simulink model "PNEUMA"  (R2023b)
settings: Solver=ode23tb  StartTime=0  StopTime=3600  FixedStep=0.001  MaxStep=time_step_new  RelTol=0.01  EnableMultiTasking=on
values from neighbouring files (symbols this model uses):
  A = 20.9    [Gas_Exchange_IC.m]    (also in getPneumonia.m = (LF1-LF2)/(1-exp(Rresolve*(t2(end)-t2(1)))))
  a1 = 0.3836    [Dissociation_Spencer_IC.m]    (also in Gas_Exchange_IC.m; Respiratory_IC.m)
  a2 = 1.819    [Dissociation_Spencer_IC.m]    (also in Gas_Exchange_IC.m; Respiratory_IC.m)
  alpha1 = 0.02598    [Dissociation_Spencer_IC.m]    (also in Gas_Exchange_IC.m; Respiratory_IC.m)
  alpha2 = 0.05591    [Dissociation_Spencer_IC.m]    (also in Gas_Exchange_IC.m; Respiratory_IC.m)
  B = 92.8    [Gas_Exchange_IC.m]    (also in getPneumonia.m = LungFunction(end)-A)
  beta1 = 0.012275    [Dissociation_Spencer_IC.m]    (also in Gas_Exchange_IC.m; Respiratory_IC.m)
  beta2 = 0.03255    [Dissociation_Spencer_IC.m]    (also in Gas_Exchange_IC.m; Respiratory_IC.m)
  C = 10570    [Gas_Exchange_IC.m]
  C1 = 9    [Dissociation_Spencer_IC.m]    (also in Gas_Exchange_IC.m; Respiratory_IC.m)
  C2 = 87.00    (= 87)    [Dissociation_Spencer_IC.m]    (also in Gas_Exchange_IC.m; Respiratory_IC.m)
  Circadian_Period = 24    [Respiratory_IC.m]    (also in State_UA_Khoo_IC.m)
  CvCO2IC = 0.5116    [Body_Khoo_IC.m]    (also in Gas_Exchange_IC.m; Respiratory_IC.m = 0.5247)
  CvO2IC = 0.1672    [Body_Khoo_IC.m]    (also in Gas_Exchange_IC.m; Respiratory_IC.m = 0.1639)
  D = -5.251    [Gas_Exchange_IC.m]
  Dead1CO2IC = 0.1020    (= 0.102)    [Dead_Space_Khoo_IC.m]    (also in Gas_Exchange_IC.m; Respiratory_IC.m = 39.5616)
  Dead1O2IC = 149.8824    [Dead_Space_Khoo_IC.m]    (also in Gas_Exchange_IC.m; Respiratory_IC.m = 104.3637)
  Dead2CO2IC = 0.5274    [Dead_Space_Khoo_IC.m]    (also in Gas_Exchange_IC.m; Respiratory_IC.m = 39.6736)
  Dead2O2IC = 149.3923    [Dead_Space_Khoo_IC.m]    (also in Gas_Exchange_IC.m; Respiratory_IC.m = 104.2258)
  Dead3CO2IC = 2.2996    [Dead_Space_Khoo_IC.m]    (also in Gas_Exchange_IC.m; Respiratory_IC.m = 39.8127)
  Dead3O2IC = 147.3503    [Dead_Space_Khoo_IC.m]    (also in Gas_Exchange_IC.m; Respiratory_IC.m = 104.0505)
  Dead4CO2IC = 8.2293    [Dead_Space_Khoo_IC.m]    (also in Gas_Exchange_IC.m; Respiratory_IC.m = 40.0061)
  Dead4O2IC = 140.5179    [Dead_Space_Khoo_IC.m]    (also in Gas_Exchange_IC.m; Respiratory_IC.m = 103.8005)
  Dead5CO2IC = 22.0757    [Dead_Space_Khoo_IC.m]    (also in Gas_Exchange_IC.m; Respiratory_IC.m = 40.3359)
  Dead5O2IC = 124.5641    [Dead_Space_Khoo_IC.m]    (also in Gas_Exchange_IC.m; Respiratory_IC.m = 103.3579)
  DtotalIC = 0.3    [NeuroMuscular_IC.m]    (also in Respiratory_IC.m = 0.32)
  E_CW = 5    [Pleural_Schuessler_IC.m]    (also in Pmus_Flow_Younes_IC.m; Resp_Mech_IC.m; Respiratory_IC.m)
  E_L = 5    [Pleural_Schuessler_IC.m]    (also in Pmus_Flow_Younes_IC.m; Resp_Mech_IC.m; Respiratory_IC.m)
  fc = 0.4/60    (= 0.00666666666667)    [Respiratory_IC.m]    (also in State_UA_Khoo_IC.m)
  fcs_max = 47.78    [Cardiovascular_IC.m]    (also in Reflex_Ursino_IC.m)
  fcs_min = 2.52    [Cardiovascular_IC.m]    (also in Reflex_Ursino_IC.m)
  fcs_zero = 25    [Respiratory_IC.m]
  FlowIC = 0    [Pmus_Flow_Younes_IC.m]    (also in Resp_Mech_IC.m; Respiratory_IC.m)
  fp_inf = 6.3    [Respiratory_IC.m]
  fp_zero = 3.2    [Respiratory_IC.m]
  fs_inf = 2.10    (= 2.1)    [Respiratory_IC.m]
  fs_zero = 16.11    [Respiratory_IC.m]
  ftbs_min = 0.1    [Cardiovascular_IC.m]    (also in SA_Node_Ursino_IC.m)
  gc = 0.008/60    (= 0.000133333333333)    [Respiratory_IC.m]    (also in State_UA_Khoo_IC.m)
  h = 0.0183    [Brain_Khoo_IC.m]    (also in Gas_Exchange_IC.m; Respiratory_IC.m)
  HP_basal = 0.58    [Cardiovascular_IC.m]    (also in SA_Node_Ursino_IC.m)
  Ic = 45    [Gas_Exchange_IC.m]    (also in Respiratory_IC.m; Vent_Drive_Khoo_IC.m)
  IpCO2 = 38    [Gas_Exchange_IC.m]    (also in Respiratory_IC.m; Vent_Drive_Khoo_IC.m)
  IpO2 = 102.4    [Gas_Exchange_IC.m]    (also in Respiratory_IC.m; Vent_Drive_Khoo_IC.m)
  K1 = 13    [Dissociation_Spencer_IC.m]    (also in Gas_Exchange_IC.m; Respiratory_IC.m)
  K2 = 194.4    [Dissociation_Spencer_IC.m]    (also in Gas_Exchange_IC.m; Respiratory_IC.m)
  k_cs = 11.758    [Cardiovascular_IC.m]    (also in Reflex_Ursino_IC.m)
  k_p = 7.06    [Respiratory_IC.m]
  k_s = 0.07    [Respiratory_IC.m]
  lambda = 863    [Gas_Exchange_IC.m]    (also in Lungs_Khoo_IC.m; Respiratory_IC.m)
  Mech_Vent_pressure = 17    [Mech_vent_test.m]
  MRbCO2 = 0.0517    [Brain_Khoo_IC.m]    (also in Gas_Exchange_IC.m; Respiratory_IC.m)
  MRCO2 = 0.0033    [Body_Khoo_IC.m]    (also in Gas_Exchange_IC.m; Respiratory_IC.m)
  MRO2 = 0.0038    [Body_Khoo_IC.m]    (also in Gas_Exchange_IC.m; Respiratory_IC.m)
  NM_block_gain = 1    [Mech_vent_test.m]
  PACO2_delayIC = 39.6041    [Cardio_Mix_Lange_IC.m]    (also in Gas_Exchange_IC.m; Respiratory_IC.m = 40.4448)
  PaCO2firstIC = 0.2150    (= 0.215)    [Cardio_Mix_Lange_IC.m]    (also in Gas_Exchange_IC.m; Respiratory_IC.m = -0.2465)
  PACO2IC = 37.1484    [Gas_Exchange_IC.m]    (also in Lungs_Khoo_IC.m; Respiratory_IC.m = 40.9432)
  PaCO2secondIC = 38.4577    [Cardio_Mix_Lange_IC.m]    (also in Gas_Exchange_IC.m; Respiratory_IC.m = 40.3928)
  PAO2_delayIC = 103.8436    [Cardio_Mix_Lange_IC.m]    (also in Gas_Exchange_IC.m; Respiratory_IC.m = 103.1223)
  PaO2firstIC = -0.2838    [Cardio_Mix_Lange_IC.m]    (also in Gas_Exchange_IC.m; Respiratory_IC.m = 0.3557)
  PAO2IC = 107.1983    [Gas_Exchange_IC.m]    (also in Lungs_Khoo_IC.m; Respiratory_IC.m = 102.5153)
  PaO2secondIC = 105.4828    [Cardio_Mix_Lange_IC.m]    (also in Gas_Exchange_IC.m; Respiratory_IC.m = 103.1435)
  PbCO2IC = 48.2858    [Brain_Khoo_IC.m]    (also in Gas_Exchange_IC.m; Respiratory_IC.m = 48.5383)
  PICO2 = 0    [Dead_Space_Khoo_IC.m]    (also in Gas_Exchange_IC.m; Respiratory_IC.m)
  PIO2 = 150    [Dead_Space_Khoo_IC.m]    (also in Gas_Exchange_IC.m; Respiratory_IC.m)
  PIO2_change = -90    [Mech_vent_test.m]    (also in Respiratory_IC.m = 0)
  Pn = 90    [Cardiovascular_IC.m]    (also in Reflex_Ursino_IC.m)
  Pt_frcIC1 = 0    [Pmus_Flow_Younes_IC.m]    (also in Resp_Mech_IC.m; Respiratory_IC.m)
  Pt_frcIC2 = 0    [Pmus_Flow_Younes_IC.m]    (also in Resp_Mech_IC.m; Respiratory_IC.m)
  QdBo = 0.8333    [Brain_Khoo_IC.m]    (also in Gas_Exchange_IC.m; Respiratory_IC.m)
  R_AW = 1.27    [Pleural_Schuessler_IC.m]    (also in Pmus_Flow_Younes_IC.m; Resp_Mech_IC.m; Respiratory_IC.m)
  R_CW = 1.03    [Pleural_Schuessler_IC.m]    (also in Pmus_Flow_Younes_IC.m; Resp_Mech_IC.m; Respiratory_IC.m)
  R_L = 1.69    [Pleural_Schuessler_IC.m]    (also in Pmus_Flow_Younes_IC.m; Resp_Mech_IC.m; Respiratory_IC.m)
  RC = 0.06    [Pleural_Schuessler_IC.m]    (also in Pmus_Flow_Younes_IC.m; Resp_Mech_IC.m; Respiratory_IC.m)
  rc = 0.2/60    (= 0.00333333333333)    [Respiratory_IC.m]    (also in State_UA_Khoo_IC.m)
  SbCO2 = 0.3600    (= 0.36)    [Brain_Khoo_IC.m]    (also in Gas_Exchange_IC.m; Respiratory_IC.m)
  SCO2 = 0.0043    [Brain_Khoo_IC.m]    (also in Gas_Exchange_IC.m; Respiratory_IC.m)
  SWAo = 0.007    [Respiratory_IC.m]    (also in State_UA_Khoo_IC.m)
  T1 = 1    [Cardio_Mix_Lange_IC.m]    (also in Gas_Exchange_IC.m; Respiratory_IC.m)
  T2 = 2    [Cardio_Mix_Lange_IC.m]    (also in Gas_Exchange_IC.m; Respiratory_IC.m)
  t_end_new = 4*24*60*60    (= 345600)    [Mech_vent_test.m]
  t_end_UA = 0    [Respiratory_IC.m]    (also in State_UA_Khoo_IC.m)
  t_Mech_Vent_duration = 0    [Mech_vent_test.m]
  t_Mech_Vent_start = 0    [Mech_vent_test.m]
  t_Mueller_duration = 0    [NeuroMuscular_IC.m]
  t_Mueller_insp = 0    [NeuroMuscular_IC.m]
  t_Mueller_start = 0    [NeuroMuscular_IC.m]
  t_NM_block_duration = 0    [Mech_vent_test.m]
  t_NM_block_start = 0    [Mech_vent_test.m]
  t_O2_duration = 0    [Mech_vent_test.m]    (also in Respiratory_IC.m)
  t_O2_start = 0    [Mech_vent_test.m]    (also in Respiratory_IC.m)
  t_start_new = 0    [Mech_vent_test.m]
  t_start_UA = 0    [Respiratory_IC.m]    (also in State_UA_Khoo_IC.m)
  t_valsalva_duration = 0    [NeuroMuscular_IC.m]
  t_valsalva_insp = 0    [NeuroMuscular_IC.m]
  t_valsalva_start = 0    [NeuroMuscular_IC.m]
  time_step = time_step    [acquire_data.m]    (also in acquire_data_save.m)
  VC = 5    [Pmus_Flow_Younes_IC.m]    (also in Resp_Mech_IC.m; Respiratory_IC.m)
  Vdead1 = 0.03    [Dead_Space_Khoo_IC.m]    (also in Gas_Exchange_IC.m; Respiratory_IC.m)
  Vdead2 = 0.03    [Dead_Space_Khoo_IC.m]    (also in Gas_Exchange_IC.m; Respiratory_IC.m)
  Vdead3 = 0.03    [Dead_Space_Khoo_IC.m]    (also in Gas_Exchange_IC.m; Respiratory_IC.m)
  Vdead4 = 0.03    [Dead_Space_Khoo_IC.m]    (also in Gas_Exchange_IC.m; Respiratory_IC.m)
  Vdead5 = 0.03    [Dead_Space_Khoo_IC.m]    (also in Gas_Exchange_IC.m; Respiratory_IC.m)
  Ventilator_rate = 12    [Mech_vent_test.m]
  VTCO2 = 15    [Body_Khoo_IC.m]    (also in Gas_Exchange_IC.m; Respiratory_IC.m)
  VtIC = 0    [Pmus_Flow_Younes_IC.m]    (also in Resp_Mech_IC.m; Respiratory_IC.m)
  VTO2 = 6    [Body_Khoo_IC.m]    (also in Gas_Exchange_IC.m; Respiratory_IC.m)
  Z = 0.0227    [Dissociation_Spencer_IC.m]    (also in Gas_Exchange_IC.m; Respiratory_IC.m)
undefined symbols (not defined in the file or in its folder): A_0_ua, alpha_E_FFA_Heart, alpha_E_FFA_muscle, alpha_E_GLC_Heart, alpha_E_GLC_muscle, alpha_E_GLY_muscle, alpha_E_PYR_muscle, alpha_E_TGL_adipose, alpha_E_TGL_GI, alpha_E_TGL_Heart, alpha_E_TGL_muscle, Arousal_UAIC, C_ua_awake, Cbp, Cbv, Ce_0, Cep, Cev, Chp, Chv, Cla, Clamp_class, Cmp, Cmv, Cpa, CPAP_pressure, Cpp, Cpv, Cra, Csa, Csp, Csv, CvbO2_n, CvhO2_n, CvmO2_n, DAY, delay, DietBlock, Dx, Fb, fchemo_max, fchemo_min, fchemoIC, flsIC, Ftas_I0, ftas_min, ftas_r0, FVC_activation, gain_E, Gamma, Gas_sleep, Gas_sleepM, Gb, Gblock, GbO2, Gbs_sleep, gcc_sa, gcc_sb, gcc_sp, Gclamp ... (+144)
libraries: simulink x4, dspstat3 x4, simulink_extras x2
(part 2 of 8)

== system PNEUMA/Cardiovascular System/Right Heart ==
  note: Right Heart
  note: Vura (Right Atrium Unstressed Volume)
      | Vurv (Right Ventricle Unstressed Volume)
      | Vrv (Right Ventricle Volume)
      | Vra (Right Atrium Volume)
      | Pra (Right Atrium Pressure)
      | Prv (Right Ventricle Pressure)
      | Qra (Flow into Right Atrium)
      | Qir (Flow into Right Ventricle)
      | Qor (Flow out of Right Ventricle)
      | LHeart (Left Ventricle Function)
  In1 : Inport
  CHF Gain : Gain
  CHF Gain1 : Gain
  Constant2 : Constant  Value=Vura
  Constant3 : Constant  Value=Vurv
  Gain : Gain  Gain=1/Cra  SaturateOnIntegerOverflow=on  OutDataTypeStr=Inherit: Same as input  ParamDataTypeStr=Inherit: Same as input
  Gain2 : Gain  Gain=1/Rra  SaturateOnIntegerOverflow=on  OutDataTypeStr=Inherit: Same as input  ParamDataTypeStr=Inherit: Same as input
  Integrator : Integrator
  Integrator1 : Integrator
  Pmaxrv--Ppa ---------------------- Rrv : Subsystem
  Product : Product  RndMeth=Zero
  SubSystem : Subsystem
  SubSystem1 : Subsystem
  Sum : Sum  Inputs=|+-  InputSameDT=on  SaturateOnIntegerOverflow=on  OutDataTypeStr=Inherit: Same as first input
  Sum1 : Sum  Inputs=|+-  InputSameDT=on  SaturateOnIntegerOverflow=on  OutDataTypeStr=Inherit: Same as first input
  Sum2 : Sum  Inputs=|++
  Sum3 : Sum  Inputs=+-  InputSameDT=on  SaturateOnIntegerOverflow=on  OutDataTypeStr=Inherit: Same as first input
  Sum4 : Sum  Inputs=+-  InputSameDT=on  SaturateOnIntegerOverflow=on  OutDataTypeStr=Inherit: Same as first input
  Sum6 : Sum  Inputs=|++
  Switch2 : Switch
  pulmonary valve : Saturate  UpperLimit=inf  LowerLimit=0
  tricuspid valve : Saturate  UpperLimit=inf  LowerLimit=0
  Out1 : Outport
  tag scope: Pra=scoped, Vra=scoped, Vrv=scoped, Wrv=scoped
  wires:
  In1/1 -> Sum/1  "Qra"
  Sum/1 -> Integrator/1
  [Ppa] -> Sum1/2
  Gain2/1 -> Sum/2, Sum4/1  "Qir"
  Integrator/1 -> SubSystem/2(+)
  Constant2/1 -> SubSystem/1(_)
  SubSystem1/1(Out) -> [Vrv]
  SubSystem/1(Out) -> Gain/1, [Vra]
  Constant3/1 -> SubSystem1/1(_)
  Integrator1/1 -> SubSystem1/2(+)
  Sum1/1 -> pulmonary valve/1, Switch2/2
  [Ppa] -> Switch2/1
  tricuspid valve/1 -> CHF Gain1/1
  pulmonary valve/1 -> Pmaxrv--Ppa ---------------------- Rrv/2(P)  "Qor"
  Pmaxrv--Ppa ---------------------- Rrv/1(Flow) -> CHF Gain/1  "Qor"
  [RHeart] -> Switch2/3, Pmaxrv--Ppa ---------------------- Rrv/1(Pmax), Sum1/1  "Pmaxrv"
  Sum4/1 -> Integrator1/1, Product/2
  Sum3/1 -> tricuspid valve/1
  Gain/1 -> Sum6/1  "Pra"
  Sum6/1 -> [Pra], Sum3/1
  Switch2/1 -> Sum2/2, Product/1  "Prv"
  Sum2/1 -> Sum3/2
  [gPpl] -> Sum2/1, Sum6/2
  Product/1 -> [Wrv]
  CHF Gain/1 -> Out1/1, Sum4/2
  CHF Gain1/1 -> Gain2/1

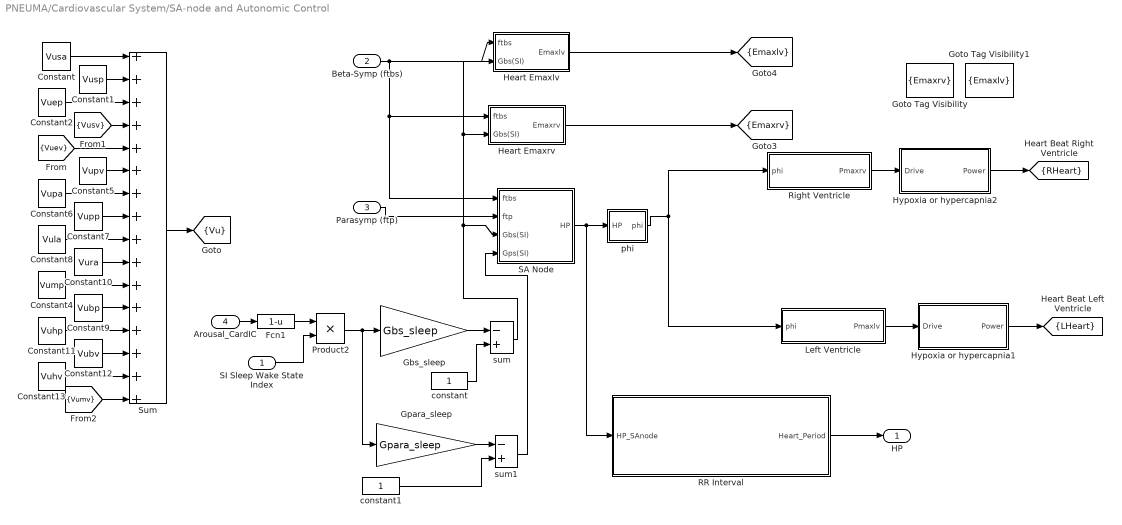
== system PNEUMA/Cardiovascular System/SA-node and Autonomic Control ==
  SI Sleep Wake State Index : Inport
  Beta-Symp (ftbs) : Inport  Port=2
  Parasymp (ftp) : Inport  Port=3
  Arousal_CardIC : Inport  Port=4
  Constant : Constant  Value=Vusa
  Constant1 : Constant  Value=Vusp
  Constant10 : Constant  Value=Vura
  Constant11 : Constant  Value=Vuhp
  Constant12 : Constant  Value=Vubv
  Constant13 : Constant  Value=Vuhv
  Constant2 : Constant  Value=Vuep
  Constant4 : Constant  Value=Vump
  Constant5 : Constant  Value=Vupv
  Constant6 : Constant  Value=Vupa
  Constant7 : Constant  Value=Vupp
  Constant8 : Constant  Value=Vula
  Constant9 : Constant  Value=Vubp
  Fcn1 : Fcn  Expr=1-u
  Gbs_sleep : Gain  Gain=Gbs_sleep  SaturateOnIntegerOverflow=on  OutDataTypeStr=Inherit: Same as input  ParamDataTypeStr=Inherit: Same as input
  Goto Tag Visibility : GotoTagVisibility  GotoTag=Emaxrv
  Goto Tag Visibility1 : GotoTagVisibility  GotoTag=Emaxlv
  Gpara_sleep : Gain  Gain=Gpara_sleep  SaturateOnIntegerOverflow=on  OutDataTypeStr=Inherit: Same as input  ParamDataTypeStr=Inherit: Same as input
  Heart Emaxlv : Subsystem
  Heart Emaxrv : Subsystem
  Hypoxia or hypercapnia1 : Subsystem
  Hypoxia or hypercapnia2 : Subsystem
  Left Ventricle : Subsystem
  Product2 : Product  InputSameDT=on  SaturateOnIntegerOverflow=on  OutDataTypeStr=Inherit: Same as first input
  RR Interval : Subsystem
  Right Ventricle : Subsystem
  SA Node : Subsystem
  Sum : Sum  Inputs=++++++++++++++++  InputSameDT=on  SaturateOnIntegerOverflow=on  OutDataTypeStr=Inherit: Same as first input
  constant : Constant
  constant1 : Constant
  phi : Subsystem
  sum : Sum  Inputs=-+  InputSameDT=on  SaturateOnIntegerOverflow=on  OutDataTypeStr=Inherit: Same as first input
  sum1 : Sum  Inputs=-+  InputSameDT=on  SaturateOnIntegerOverflow=on  OutDataTypeStr=Inherit: Same as first input
  HP : Outport
  tag scope: Emaxlv=scoped, Emaxrv=scoped, LHeart=scoped, RHeart=scoped, Vu=scoped
  wires:
  Arousal_CardIC/1 -> Fcn1/1
  SI Sleep Wake State Index/1 -> Product2/2
  sum/1 -> Heart Emaxrv/2(Gbs(SI)), Heart Emaxlv/2(Gbs(SI)), SA Node/3(Gbs(SI))
  sum1/1 -> SA Node/4(Gps(SI))
  Fcn1/1 -> Product2/1
  Product2/1 -> Gbs_sleep/1, Gpara_sleep/1
  Gbs_sleep/1 -> sum/1
  constant/1 -> sum/2
  Gpara_sleep/1 -> sum1/1
  constant1/1 -> sum1/2
  Sum/1 -> [Vu]
  Constant/1 -> Sum/1
  Constant2/1 -> Sum/3
  Constant1/1 -> Sum/2
  [Vusv] -> Sum/4
  [Vuev] -> Sum/5
  Constant5/1 -> Sum/6
  Constant6/1 -> Sum/7
  Constant7/1 -> Sum/8
  Constant8/1 -> Sum/9
  Constant10/1 -> Sum/10
  Constant4/1 -> Sum/11
  Constant9/1 -> Sum/12
  Constant11/1 -> Sum/13
  Constant12/1 -> Sum/14
  Constant13/1 -> Sum/15
  [Vumv] -> Sum/16
  phi/1(phi) -> Right Ventricle/1(phi), Left Ventricle/1(phi)
  SA Node/1(HP) -> phi/1(HP), RR Interval/1(HP_SAnode)
  Beta-Symp (ftbs)/1 -> Heart Emaxrv/1(ftbs), SA Node/1(ftbs), Heart Emaxlv/1(ftbs)
  Parasymp (ftp)/1 -> SA Node/2(ftp)
  RR Interval/1(Heart_Period) -> HP/1
  Heart Emaxlv/1(Emaxlv) -> [Emaxlv]
  Heart Emaxrv/1(Emaxrv) -> [Emaxrv]
  Left Ventricle/1(Pmaxlv) -> Hypoxia or hypercapnia1/1(Drive)
  Hypoxia or hypercapnia1/1(Power) -> [LHeart]
  Right Ventricle/1(Pmaxrv) -> Hypoxia or hypercapnia2/1(Drive)
  Hypoxia or hypercapnia2/1(Power) -> [RHeart]

== system PNEUMA/Cardiovascular System/Systemic ==
  note: Psa (Systemic Arteries Pressure)
      | Psp (Splanchnic Peripheral Pressure)
      | Pep (Extrasplanchnic Peripheral Pressure)
      | Psv (Splanchnic Venous Pressure)
      | Pvc (Vena Cava Pressure)
      | Pra (Right Atrium Pressure)
      | For (Flow from Left Heart)
      | Fsa (Flow to Systemic Aorta)
      | Fil (Flow to Left Atrium)
      | Fvc (Flow to Vena Cava)
      | Fra (Flow to Right Atrium)
      | Vusa (Systemic Arteries Unstressed Volume)
      | Vusp (Extrasplanchnic Venous Unstressed Volume)
      | Vuep (Splanchnic Venous Unstressed Volume)
      | Vuev (Extrasplanchnic Venous Unstressed Volume)
      | Vusv (Splanchnic Venous Unstressed Volume)
  note: Systemic Circulation
  Qlv : Inport
  Goto Tag Visibility7 : GotoTagVisibility  GotoTag=Vvc
  Systemic Arteries : Subsystem
  Systemic Peripheral & Venous Circulation : Subsystem
  Vena Cava : Subsystem
  Qra : Outport
  Qmp : Outport  Port=2
  Qbp : Outport  Port=3
  Qhp : Outport  Port=4
  wires:
  Qlv/1 -> Systemic Arteries/1(Qlv)  "Fol"
  Systemic Arteries/1(Qsa) -> Systemic Peripheral & Venous Circulation/1(Qsa)
  Vena Cava/1(Qra) -> Qra/1
  Systemic Peripheral & Venous Circulation/1(Qvc) -> Vena Cava/1(Qvc)
  Systemic Peripheral & Venous Circulation/2(Qmp) -> Qmp/1
  Systemic Peripheral & Venous Circulation/3(Qbp) -> Qbp/1
  Systemic Peripheral & Venous Circulation/4(Qhp) -> Qhp/1

== system PNEUMA/Cardiovascular System/TPR Change ==
  Alpha Symp (ftas) : Inport
  Alpha Symp (ftas_vein) : Inport  Port=2
  AI (arousal  Index) : Inport  Port=3
  "SI (Sleep Index) " : Inport  Port=4
  Fcn1 : Fcn  Expr=1-u
  Gas_sleep : Gain  Gain=Gas_sleep  SaturateOnIntegerOverflow=on  OutDataTypeStr=Inherit: Same as input  ParamDataTypeStr=Inherit: Same as input
  Math Function{,1..4} (5 alike) : Math  Operator=reciprocal  SignedPower=on
  Mux : Mux  Inputs=10
  Peri Circ Rep : Subsystem
  Peri Circ Rmp : Subsystem
  Peri Circ Rsp : Subsystem
  Product2 : Product  InputSameDT=on  SaturateOnIntegerOverflow=on  OutDataTypeStr=Inherit: Same as first input
  Saving TPR : Subsystem
  Sum1 : Sum  Inputs=+++++  InputSameDT=on  SaturateOnIntegerOverflow=on  OutDataTypeStr=Inherit: Same as first input
  Sum3 : Sum  Inputs=-+  InputSameDT=on  SaturateOnIntegerOverflow=on  OutDataTypeStr=Inherit: Same as first input
  Venous Circ Vuev : Subsystem
  Venous Circ Vumv : Subsystem
  Venous Circ Vusv : Subsystem
  constant : Constant
  tag scope: Rep=scoped, Rmpn=scoped, Rsp=scoped, TPR_change=global, Vuev=scoped, Vumv=scoped, Vusv=scoped
  wires:
  AI (arousal  Index)/1 -> Fcn1/1
  "SI (Sleep Index) "/1 -> Product2/2
  Fcn1/1 -> Product2/1
  Product2/1 -> Gas_sleep/1
  constant/1 -> Sum3/2
  Gas_sleep/1 -> Sum3/1
  Peri Circ Rep/1(Rep) -> [Rep], Math Function1/1, Mux/2  "Rep"
  Venous Circ Vusv/1(Vusv) -> [Vusv], Mux/7  "Vusv"
  Venous Circ Vuev/1(Vuev) -> [Vuev], Mux/8  "Vuev"
  Peri Circ Rsp/1(Rsp) -> [Rsp], Math Function/1, Mux/1  "Rsp"
  Venous Circ Vumv/1(Vumv) -> [Vumv], Mux/9  "Vumv"
  Peri Circ Rmp/1(Rmp_n) -> [Rmpn], Mux/3  "Rmp_n"
  Alpha Symp (ftas)/1 -> Peri Circ Rep/1(fes), Peri Circ Rmp/1(fes), Peri Circ Rsp/1(fes)
  Sum3/1 -> Peri Circ Rsp/2(Gas(SI)), Peri Circ Rep/2(Gas(SI)), Venous Circ Vusv/2(Gas(SI)), Venous Circ Vuev/2(Gas(SI)), Venous Circ Vumv/2(Gas(SI)), Peri Circ Rmp/2(Gas(SI))  "Gas(SI)"
  Alpha Symp (ftas_vein)/1 -> Venous Circ Vusv/1(fes), Venous Circ Vuev/1(fes), Venous Circ Vumv/1(fes)
  Sum1/1 -> Math Function4/1
  [Gbp] -> Sum1/3, Mux/4  "Gbp"
  [Rmp] -> Math Function2/1, Mux/5  "Rmp"
  [Rhp] -> Math Function3/1, Mux/6  "Rhp"
  Math Function/1 -> Sum1/1
  Math Function1/1 -> Sum1/2
  Math Function2/1 -> Sum1/4
  Math Function3/1 -> Sum1/5
  Math Function4/1 -> [TPR_change], Mux/10
  Mux/1 -> Saving TPR/1(In1)

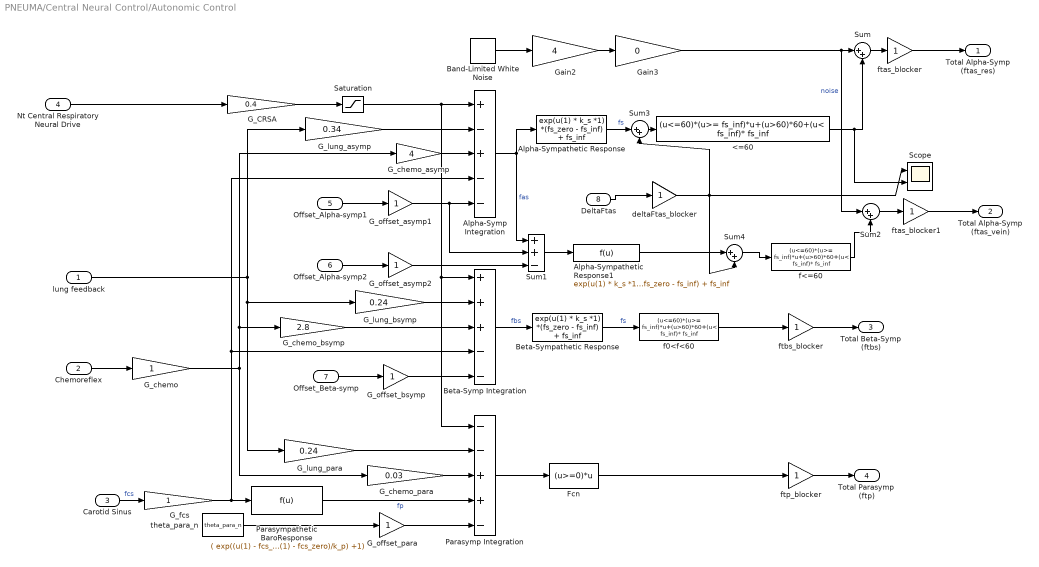
== system PNEUMA/Central Neural Control/Autonomic Control ==
  lung feedback : Inport
  Chemoreflex : Inport  Port=2
  Carotid Sinus : Inport  Port=3
  Nt Central Respiratory Neural Drive : Inport  Port=4
  Offset_Alpha-symp1 : Inport  Port=5
  Offset_Alpha-symp2 : Inport  Port=6
  Offset_Beta-symp : Inport  Port=7
  DeltaFtas : Inport  Port=8
  <=60 : Fcn  Expr=(u<=60)*(u>= fs_inf)*u+(u>60)*60+(u< fs_inf)* fs_inf
  Alpha-Symp Integration : Sum  Inputs=+-+--  InputSameDT=on  SaturateOnIntegerOverflow=on  OutDataTypeStr=Inherit: Same as first input
  Alpha-Sympathetic Response : Fcn  Expr=exp(u(1) * k_s *1) *(fs_zero - fs_inf) + fs_inf
  Alpha-Sympathetic Response1 : Fcn  Expr=exp(u(1) * k_s *1) *(fs_zero - fs_inf) + fs_inf
  Band-Limited White Noise : simulink/Sources/Band-Limited White Noise  Cov=[0.025]  Ts=0.1  seed=[23341]
  Beta-Symp Integration : Sum  Inputs=+++--  InputSameDT=on  SaturateOnIntegerOverflow=on  OutDataTypeStr=Inherit: Same as first input
  Beta-Sympathetic Response : Fcn  Expr=exp(u(1) * k_s *1) *(fs_zero - fs_inf) + fs_inf
  Fcn : Fcn  Expr=(u>=0)*u
  G_CRSA : Gain  Gain=0.4  SaturateOnIntegerOverflow=on  OutDataTypeStr=Inherit: Same as input  ParamDataTypeStr=Inherit: Same as input
  G_chemo : Gain  SaturateOnIntegerOverflow=on  OutDataTypeStr=Inherit: Same as input  ParamDataTypeStr=Inherit: Same as input
  G_chemo_asymp : Gain  Gain=4  SaturateOnIntegerOverflow=on  OutDataTypeStr=Inherit: Same as input  ParamDataTypeStr=Inherit: Same as input
  G_chemo_bsymp : Gain  Gain=2.8  SaturateOnIntegerOverflow=on  OutDataTypeStr=Inherit: Same as input  ParamDataTypeStr=Inherit: Same as input
  G_chemo_para : Gain  Gain=0.03  SaturateOnIntegerOverflow=on  OutDataTypeStr=Inherit: Same as input  ParamDataTypeStr=Inherit: Same as input
  G_fcs : Gain  SaturateOnIntegerOverflow=on  OutDataTypeStr=Inherit: Same as input  ParamDataTypeStr=Inherit: Same as input
  G_lung_asymp : Gain  Gain=0.34  SaturateOnIntegerOverflow=on  OutDataTypeStr=Inherit: Same as input  ParamDataTypeStr=Inherit: Same as input
  G_lung_bsymp : Gain  Gain=0.24  SaturateOnIntegerOverflow=on  OutDataTypeStr=Inherit: Same as input  ParamDataTypeStr=Inherit: Same as input
  G_lung_para : Gain  Gain=0.24  SaturateOnIntegerOverflow=on  OutDataTypeStr=Inherit: Same as input  ParamDataTypeStr=Inherit: Same as input
  G_offset_asymp1 : Gain
  G_offset_asymp2 : Gain
  G_offset_bsymp : Gain
  G_offset_para : Gain
  Gain2 : Gain  Gain=4  SaturateOnIntegerOverflow=on  OutDataTypeStr=Inherit: Same as input  ParamDataTypeStr=Inherit: Same as input
  Gain3 : Gain  Gain=0  SaturateOnIntegerOverflow=on  OutDataTypeStr=Inherit: Same as input  ParamDataTypeStr=Inherit: Same as input
  "Parasymp Integration " : Sum  Inputs=--++-  InputSameDT=on  SaturateOnIntegerOverflow=on  OutDataTypeStr=Inherit: Same as first input
  Parasympathetic BaroResponse : Fcn  Expr=( exp((u(1) - fcs_zero)/k_p) * fp_inf *1 + fp_zero) / (exp((u(1) - fcs_zero)/k_p) +1)
  Saturation : Saturate  UpperLimit=10  LowerLimit=-10
  Scope : Scope  NumInputPorts=2
  Sum{,2..4} (4 alike) : Sum  Inputs=|++  SaturateOnIntegerOverflow=on
  Sum1 : Sum  Inputs=++-  SaturateOnIntegerOverflow=on
  deltaFtas_blocker : Gain  SaturateOnIntegerOverflow=on  OutDataTypeStr=Inherit: Same as input  ParamDataTypeStr=Inherit: Same as input
  f0<f<60 : Fcn  Expr=(u<=60)*(u>= fs_inf)*u+(u>60)*60+(u< fs_inf)* fs_inf
  f<=60 : Fcn  Expr=(u<=60)*(u>= fs_inf)*u+(u>60)*60+(u< fs_inf)* fs_inf
  ftas_blocker : Gain  SaturateOnIntegerOverflow=on  OutDataTypeStr=Inherit: Same as input  ParamDataTypeStr=Inherit: Same as input
  ftas_blocker1 : Gain  SaturateOnIntegerOverflow=on  OutDataTypeStr=Inherit: Same as input  ParamDataTypeStr=Inherit: Same as input
  ftbs_blocker : Gain  SaturateOnIntegerOverflow=on  OutDataTypeStr=Inherit: Same as input  ParamDataTypeStr=Inherit: Same as input
  ftp_blocker : Gain  SaturateOnIntegerOverflow=on  OutDataTypeStr=Inherit: Same as input  ParamDataTypeStr=Inherit: Same as input
  theta_para_n : Constant  Value=theta_para_n
  Total Alpha-Symp (ftas_res) : Outport
  Total Alpha-Symp (ftas_vein) : Outport  Port=2
  Total Beta-Symp (ftbs) : Outport  Port=3
  Total Parasymp (ftp) : Outport  Port=4
  wires:
  G_CRSA/1 -> Saturation/1
  Carotid Sinus/1 -> G_fcs/1  "fcs"
  "Parasymp Integration "/1 -> Fcn/1
  Beta-Symp Integration/1 -> Beta-Sympathetic Response/1  "fbs"
  lung feedback/1 -> G_lung_para/1, G_lung_bsymp/1, G_lung_asymp/1
  Chemoreflex/1 -> G_chemo/1
  Alpha-Symp Integration/1 -> Alpha-Sympathetic Response/1, Sum1/1  "fas"
  Fcn/1 -> ftp_blocker/1
  Beta-Sympathetic Response/1 -> f0<f<60/1  "fs"
  Nt Central Respiratory Neural Drive/1 -> G_CRSA/1
  Parasympathetic BaroResponse/1 -> "Parasymp Integration "/4  "fp"
  G_chemo_para/1 -> "Parasymp Integration "/3
  G_lung_para/1 -> "Parasymp Integration "/2
  G_chemo_bsymp/1 -> Beta-Symp Integration/3
  G_lung_bsymp/1 -> Beta-Symp Integration/2
  G_lung_asymp/1 -> Alpha-Symp Integration/2
  G_chemo_asymp/1 -> Alpha-Symp Integration/3
  Band-Limited White Noise/1 -> Gain2/1
  Gain2/1 -> Gain3/1
  Gain3/1 -> Sum/1, Sum2/1  "noise"
  Sum/1 -> ftas_blocker/1
  f0<f<60/1 -> ftbs_blocker/1
  <=60/1 -> Sum/2, Scope/2
  ftas_blocker/1 -> Total Alpha-Symp (ftas_res)/1
  ftbs_blocker/1 -> Total Beta-Symp (ftbs)/1
  ftp_blocker/1 -> Total Parasymp (ftp)/1
  Saturation/1 -> Alpha-Symp Integration/1, "Parasymp Integration "/1, Beta-Symp Integration/1
  G_fcs/1 -> Alpha-Symp Integration/4, Beta-Symp Integration/4, Parasympathetic BaroResponse/1
  Offset_Alpha-symp1/1 -> G_offset_asymp1/1
  Offset_Beta-symp/1 -> G_offset_bsymp/1
  theta_para_n/1 -> G_offset_para/1
  Offset_Alpha-symp2/1 -> G_offset_asymp2/1
  f<=60/1 -> Sum2/2
  Sum2/1 -> ftas_blocker1/1
  ftas_blocker1/1 -> Total Alpha-Symp (ftas_vein)/1
  Sum1/1 -> Alpha-Sympathetic Response1/1
  G_offset_asymp1/1 -> Sum1/2, Alpha-Symp Integration/5
  G_offset_asymp2/1 -> Sum1/3
  G_offset_bsymp/1 -> Beta-Symp Integration/5
  G_offset_para/1 -> "Parasymp Integration "/5
  G_chemo/1 -> G_chemo_para/1, G_chemo_asymp/1, G_chemo_bsymp/1
  Alpha-Sympathetic Response/1 -> Sum3/1  "fs"
  Sum3/1 -> <=60/1
  Alpha-Sympathetic Response1/1 -> Sum4/1
  Sum4/1 -> f<=60/1
  DeltaFtas/1 -> deltaFtas_blocker/1
  deltaFtas_blocker/1 -> Sum3/2, Sum4/2, Scope/1

== system PNEUMA/Central Neural Control/CNS response ==
  PaO2 : Inport
  PaCO2 : Inport  Port=2
  1/tao_cc : Gain  Gain=1/tao_cc
  1/tao_cc1 : Gain  Gain=1/tao_cc
  1/tao_cc2 : Gain  Gain=1/tao_cc
  1/tao_isc : Gain  Gain=1/tao_isc
  1/tao_isc1 : Gain  Gain=1/tao_isc
  1/tao_isc2 : Gain  Gain=1/tao_isc
  Gain1 : Gain  Gain=gcc_sp*0
  Gain2 : Gain  Gain=gcc_sa*0.7
  Gain3 : Gain  Gain=gcc_sb
  Integrator{,1..5} (6 alike) : Integrator
  PaCO2_n : Constant  Value=PaCO2_n
  Sum{,1..2,4..5,7..8} (7 alike) : Sum  Inputs=+-  InputSameDT=on  SaturateOnIntegerOverflow=on  OutDataTypeStr=Inherit: Same as first input
  Sum3 : Sum  Inputs=+--  InputSameDT=on  SaturateOnIntegerOverflow=on  OutDataTypeStr=Inherit: Same as first input
  Sum6 : Sum  Inputs=+--  InputSameDT=on  SaturateOnIntegerOverflow=on  OutDataTypeStr=Inherit: Same as first input
  Sum9 : Sum  Inputs=+--  InputSameDT=on  SaturateOnIntegerOverflow=on  OutDataTypeStr=Inherit: Same as first input
  Wsa_Fcn : Fcn  Expr=Xsa/(1 + exp((u - hatPO2_sa)/k_isc_sa ))
  Wsb_Fcn2 : Fcn  Expr=Xsb/(1 + exp((u - hatPO2_sb)/k_isc_sb ))
  Wsp_Fcn1 : Fcn  Expr=Xsp/(1 + exp((u - hatPO2_sp)/k_isc_sp ))
  theta_sa_n : Constant  Value=theta_sa_n
  theta_sb_n : Constant  Value=theta_sb_n
  theta_sp_n : Constant  Value=theta_sp_n
  Offset_Resistance : Outport
  Offset_veins : Outport  Port=2
  Offset_heart : Outport  Port=3
  wires:
  PaO2/1 -> Wsa_Fcn/1, Wsp_Fcn1/1, Wsb_Fcn2/1
  1/tao_isc/1 -> Integrator/1
  Integrator/1 -> Sum/2, Sum3/2  "theta_O2_sa"
  Wsa_Fcn/1 -> Sum/1
  Sum/1 -> 1/tao_isc/1
  1/tao_cc/1 -> Integrator1/1
  Integrator1/1 -> Sum1/2, Sum3/3  "theta_CO2_sa"
  Sum2/1 -> Gain2/1, Gain1/1, Gain3/1
  Sum1/1 -> 1/tao_cc/1
  PaCO2/1 -> Sum2/1
  PaCO2_n/1 -> Sum2/2
  Gain2/1 -> Sum1/1
  theta_sa_n/1 -> Sum3/1
  Sum3/1 -> Offset_Resistance/1
  1/tao_isc1/1 -> Integrator2/1
  Integrator2/1 -> Sum4/2, Sum6/2  "theta_O2_sp"
  Wsp_Fcn1/1 -> Sum4/1
  Sum4/1 -> 1/tao_isc1/1
  1/tao_cc1/1 -> Integrator3/1
  Integrator3/1 -> Sum5/2, Sum6/3  "theta_CO2_sp"
  Sum5/1 -> 1/tao_cc1/1
  Gain1/1 -> Sum5/1
  theta_sp_n/1 -> Sum6/1
  Sum6/1 -> Offset_veins/1
  1/tao_isc2/1 -> Integrator4/1
  Integrator4/1 -> Sum7/2, Sum9/2  "theta_O2_sb"
  Wsb_Fcn2/1 -> Sum7/1
  Sum7/1 -> 1/tao_isc2/1
  1/tao_cc2/1 -> Integrator5/1
  Integrator5/1 -> Sum8/2, Sum9/3  "theta_CO2_sb"
  Sum8/1 -> 1/tao_cc2/1
  Gain3/1 -> Sum8/1
  theta_sb_n/1 -> Sum9/1
  Sum9/1 -> Offset_heart/1

== system PNEUMA/Central Neural Control/Hypoxia or hypercapnia ==
  Drive : Inport
  Divide : Product  Inputs=**
  Power : Outport
  wires:
  [MuscleContractility] -> Divide/1
  Divide/1 -> Power/1  "muscle power"
  Drive/1 -> Divide/2  "Muscle drive"

== system PNEUMA/Central Neural Control/Maneuvers' Modification ==
  note: !!Add more effort for Insp
  Constant : Constant  Value=0
  Fcn1 : Fcn  Expr=(u(1)==0)*u(1)+(u(1)==1)*u(2)
  Fcn2 : Fcn  Expr=(u(1)==0)*u(1)+(u(1)==1)*u(2)
  Fcn4 : Fcn  Expr=(u(1)==0)*u(1)+(u(1)==1)*u(2)*1
  Gain : Gain  Gain=-1/1.2
  Gain1 : Gain  Gain=-1
  Gain2 : Gain
  Gain3 : Gain
  Integrator : Integrator  ExternalReset=rising  InitialCondition=-1.6
  Mux1 : Mux  Inputs=2
  Mux5 : Mux  Inputs=2
  Mux6 : Mux  Inputs=2
  Product1 : Product  RndMeth=Zero
  Product2 : Product  RndMeth=Zero
  Product4 : Product  RndMeth=Zero
  Ramp1 : simulink/Sources/Ramp  slope=0.5  start=t_FVC_start  InitialOutput=0
  Ramp2 : simulink/Sources/Ramp  slope=-0.5  start=t_FVC_start + t_FVC_insp  InitialOutput=1
  Sum : Sum  Inputs=+-
  Sum1 : Sum  Inputs=+--  InputSameDT=on  SaturateOnIntegerOverflow=on  OutDataTypeStr=Inherit: Same as first input
  Modified Nt : Outport
  wires:
  Mux5/1 -> Fcn4/1
  [FVC_activation] -> Mux5/1
  [FVC_resp_mech] -> Mux5/2
  Mux6/1 -> Fcn1/1
  [Valsalva_activation] -> Mux6/1
  [Valsalva_resp_mech] -> Mux6/2, Integrator/2
  Sum1/1 -> Modified Nt/1
  Mux1/1 -> Fcn2/1
  [FVC_activation] -> Mux1/1
  [FVC_resp_rhythm] -> Mux1/2
  Fcn2/1 -> Product1/1
  Ramp1/1 -> Product1/2
  Product1/1 -> Sum1/1
  Fcn4/1 -> Product2/1
  Product2/1 -> Gain2/1
  Ramp2/1 -> Product2/2
  Fcn1/1 -> Product4/1
  Product4/1 -> Gain3/1
  Integrator/1 -> Sum/1, Gain1/1
  Sum/1 -> Gain/1
  Gain/1 -> Integrator/1
  Constant/1 -> Sum/2
  Gain1/1 -> Product4/2
  Gain3/1 -> Sum1/3
  Gain2/1 -> Sum1/2

== system PNEUMA/Central Neural Control/Modified Resp Rhythm ==
  Resp Rhythm : Inport
  Demux : Demux  Outputs=3
      settings: DisplayOption=none
  Fcn1 : Fcn  Expr=1+u
  Fcn2 : Fcn  Expr=(u(1)==0)*1+(u(1)==1)*u(2)
  Fcn3 : Fcn  Expr=(u(1)==0)*1+(u(1)==1)*u(2)
  Fcn4 : Fcn  Expr=(u(1)==0)*1+(u(1)==1)*u(2)
  Mux1 : Mux  Inputs=2
  Mux2 : Mux  Inputs=2
  Mux3 : Mux  Inputs=2
  Product1 : Product  Inputs=*****  InputSameDT=on  SaturateOnIntegerOverflow=on  OutDataTypeStr=Inherit: Same as first input
  Res Rhythm : Scope  NumInputPorts=2
  Sum3 : Sum  Inputs=++++  InputSameDT=on  SaturateOnIntegerOverflow=on  OutDataTypeStr=Inherit: Same as first input
  Terminator : Terminator
  Terminator3 : Terminator
  "modified resp rhythm " : Outport
  wires:
  Fcn1/1 -> Product1/5
  [upper_airway_blockage_duration] -> Fcn1/1
  Sum3/1 -> Res Rhythm/2, Demux/1
  Product1/1 -> Sum3/4
  [Mueller_resp_rhythm] -> Sum3/1
  Resp Rhythm/1 -> Product1/1, Res Rhythm/1
  [Mueller_duration] -> Mux3/2
  [Mueller_activation] -> Mux3/1
  Mux3/1 -> Fcn2/1
  Fcn2/1 -> Product1/2
  [Valsalva_activation] -> Mux1/1
  [Valsalva_duration] -> Mux1/2
  Mux1/1 -> Fcn3/1
  Fcn3/1 -> Product1/3
  [Valsalva_resp_rhythm] -> Sum3/2
  [FVC_resp_rhythm] -> Sum3/3
  [FVC_activation] -> Mux2/1
  [FVC_duration] -> Mux2/2
  Mux2/1 -> Fcn4/1
  Fcn4/1 -> Product1/4
  Demux/3 -> Terminator3/1
  Demux/1 -> Terminator/1
  Demux/2 -> "modified resp rhythm "/1

== system PNEUMA/Central Neural Control/Nt Save block ==
  Resp_sig : Inport
  Fcn1 : Fcn  Expr=u(1)*u(2)
  Fcn2 : Fcn  Expr=u(1)
  Integrator : Integrator  ExternalReset=falling  AbsoluteTolerance=0.00000000001
  Nt Saturation : Saturate  UpperLimit=10  LowerLimit=0  ZeroCross=off
  Nt Central Respiratory Neural Drive : Outport
  tag scope: Nt=global
  wires:
  Fcn2/1 -> Integrator/2
  Fcn1/1 -> Integrator/1
  Resp_sig/1 -> Fcn1/1, Fcn2/1
  Integrator/1 -> [Nt], Nt Saturation/1
  Nt Saturation/1 -> Nt Central Respiratory Neural Drive/1

== system PNEUMA/Central Neural Control/Saving AutonomicCtrl ==
  In1 : Inport
  Clock : Clock
  Gain : Gain  Gain=1/(3600*24*DAY)
  Rounding Function : Rounding
  Switch Case : SwitchCase  CaseConditions={0,1,2,3,4,5,6,7,8}  SampleTime=sampletime
  Switch Case Action Subsystem : Subsystem  TreatAsAtomicUnit=on
  Switch Case Action Subsystem1 : Subsystem  TreatAsAtomicUnit=on
  Switch Case Action Subsystem2 : Subsystem  TreatAsAtomicUnit=on
  Switch Case Action Subsystem3 : Subsystem  TreatAsAtomicUnit=on
  Switch Case Action Subsystem4 : Subsystem  TreatAsAtomicUnit=on
  Switch Case Action Subsystem5 : Subsystem  TreatAsAtomicUnit=on
  Switch Case Action Subsystem6 : Subsystem  TreatAsAtomicUnit=on
  Switch Case Action Subsystem7 : Subsystem  TreatAsAtomicUnit=on
  Switch Case Action Subsystem8 : Subsystem  TreatAsAtomicUnit=on
  Switch Case Action Subsystem9 : Subsystem  TreatAsAtomicUnit=on
  wires:
  Clock/1 -> Gain/1
  Switch Case/1 -> Switch Case Action Subsystem/Action
  Switch Case/2 -> Switch Case Action Subsystem1/Action
  Switch Case/3 -> Switch Case Action Subsystem2/Action
  Switch Case/10 -> Switch Case Action Subsystem3/Action
  Rounding Function/1 -> Switch Case/1
  In1/1 -> Switch Case Action Subsystem/1(In1), Switch Case Action Subsystem1/1(In1), Switch Case Action Subsystem2/1(In1), Switch Case Action Subsystem4/1(In1), Switch Case Action Subsystem5/1(In1), Switch Case Action Subsystem3/1(In1), Switch Case Action Subsystem9/1(In1), Switch Case Action Subsystem8/1(In1), Switch Case Action Subsystem7/1(In1), Switch Case Action Subsystem6/1(In1)
  Gain/1 -> Rounding Function/1
  Switch Case/4 -> Switch Case Action Subsystem4/Action
  Switch Case/5 -> Switch Case Action Subsystem5/Action
  Switch Case/6 -> Switch Case Action Subsystem6/Action
  Switch Case/7 -> Switch Case Action Subsystem7/Action
  Switch Case/8 -> Switch Case Action Subsystem8/Action
  Switch Case/9 -> Switch Case Action Subsystem9/Action

== system PNEUMA/Central Neural Control/Saving Nt ==
  In1 : Inport
  Clock : Clock
  Gain : Gain  Gain=1/(3600*24*DAY)
  Rounding Function : Rounding
  Switch Case : SwitchCase  CaseConditions={0,1,2,3,4,5,6,7,8}  SampleTime=sampletime
  Switch Case Action Subsystem : Subsystem  TreatAsAtomicUnit=on
  Switch Case Action Subsystem1 : Subsystem  TreatAsAtomicUnit=on
  Switch Case Action Subsystem2 : Subsystem  TreatAsAtomicUnit=on
  Switch Case Action Subsystem3 : Subsystem  TreatAsAtomicUnit=on
  Switch Case Action Subsystem4 : Subsystem  TreatAsAtomicUnit=on
  Switch Case Action Subsystem5 : Subsystem  TreatAsAtomicUnit=on
  Switch Case Action Subsystem6 : Subsystem  TreatAsAtomicUnit=on
  Switch Case Action Subsystem7 : Subsystem  TreatAsAtomicUnit=on
  Switch Case Action Subsystem8 : Subsystem  TreatAsAtomicUnit=on
  Switch Case Action Subsystem9 : Subsystem  TreatAsAtomicUnit=on
  wires:
  Clock/1 -> Gain/1
  Switch Case/1 -> Switch Case Action Subsystem/Action
  Switch Case/2 -> Switch Case Action Subsystem1/Action
  Switch Case/3 -> Switch Case Action Subsystem2/Action
  Switch Case/10 -> Switch Case Action Subsystem3/Action
  Rounding Function/1 -> Switch Case/1
  In1/1 -> Switch Case Action Subsystem/1(In1), Switch Case Action Subsystem1/1(In1), Switch Case Action Subsystem2/1(In1), Switch Case Action Subsystem4/1(In1), Switch Case Action Subsystem5/1(In1), Switch Case Action Subsystem3/1(In1), Switch Case Action Subsystem9/1(In1), Switch Case Action Subsystem8/1(In1), Switch Case Action Subsystem7/1(In1), Switch Case Action Subsystem6/1(In1)
  Gain/1 -> Rounding Function/1
  Switch Case/4 -> Switch Case Action Subsystem4/Action
  Switch Case/5 -> Switch Case Action Subsystem5/Action
  Switch Case/6 -> Switch Case Action Subsystem6/Action
  Switch Case/7 -> Switch Case Action Subsystem7/Action
  Switch Case/8 -> Switch Case Action Subsystem8/Action
  Switch Case/9 -> Switch Case Action Subsystem9/Action

== system PNEUMA/Central Neural Control/Saving Resp_Rhythm ==
  In1 : Inport
  Clock : Clock
  Gain : Gain  Gain=1/(3600*24*DAY)
  Rounding Function : Rounding
  Switch Case : SwitchCase  CaseConditions={0,1,2,3,4,5,6,7,8}  SampleTime=sampletime
  Switch Case Action Subsystem : Subsystem  TreatAsAtomicUnit=on
  Switch Case Action Subsystem1 : Subsystem  TreatAsAtomicUnit=on
  Switch Case Action Subsystem2 : Subsystem  TreatAsAtomicUnit=on
  Switch Case Action Subsystem3 : Subsystem  TreatAsAtomicUnit=on
  Switch Case Action Subsystem4 : Subsystem  TreatAsAtomicUnit=on
  Switch Case Action Subsystem5 : Subsystem  TreatAsAtomicUnit=on
  Switch Case Action Subsystem6 : Subsystem  TreatAsAtomicUnit=on
  Switch Case Action Subsystem7 : Subsystem  TreatAsAtomicUnit=on
  Switch Case Action Subsystem8 : Subsystem  TreatAsAtomicUnit=on
  Switch Case Action Subsystem9 : Subsystem  TreatAsAtomicUnit=on
  wires:
  Clock/1 -> Gain/1
  Switch Case/1 -> Switch Case Action Subsystem/Action
  Switch Case/2 -> Switch Case Action Subsystem1/Action
  Switch Case/3 -> Switch Case Action Subsystem2/Action
  Switch Case/10 -> Switch Case Action Subsystem3/Action
  Rounding Function/1 -> Switch Case/1
  In1/1 -> Switch Case Action Subsystem/1(In1), Switch Case Action Subsystem1/1(In1), Switch Case Action Subsystem2/1(In1), Switch Case Action Subsystem5/1(In1), Switch Case Action Subsystem3/1(In1), Switch Case Action Subsystem9/1(In1), Switch Case Action Subsystem8/1(In1), Switch Case Action Subsystem7/1(In1), Switch Case Action Subsystem6/1(In1), Switch Case Action Subsystem4/1(In1)
  Gain/1 -> Rounding Function/1
  Switch Case/4 -> Switch Case Action Subsystem4/Action
  Switch Case/5 -> Switch Case Action Subsystem5/Action
  Switch Case/6 -> Switch Case Action Subsystem6/Action
  Switch Case/7 -> Switch Case Action Subsystem7/Action
  Switch Case/8 -> Switch Case Action Subsystem8/Action
  Switch Case/9 -> Switch Case Action Subsystem9/Action

== system PNEUMA/Central Neural Control/VARIABLE RESPIRATORY RHYTHM1 ==
  D_Total : Inport
  60*TI/TT : Gain  Gain=22.5  SaturateOnIntegerOverflow=on  OutDataTypeStr=Inherit: Same as input  ParamDataTypeStr=Inherit: Same as input
  Enable Breathing Signal : Subsystem
  Gain : Gain  Gain=60
  Math Function : Math  Operator=reciprocal  SignedPower=on
  Respiratory Rhythm_Generator : Subsystem  TreatAsAtomicUnit=on
  VBF_fcn : Fcn  Expr=(u<V_b)*F_b+(u>V_P)*(S1_F*(T_P-T_D)+S2_F*(u-S1_V*(T_P-T_D)-V_b)/S2_V+F_b)+(u>=V_b)*(u<=V_P)*(S1_F*(u- V_b)/S1_V+F_b)
  Variable Breathing Period Reset : Subsystem
  Ventilator override : Subsystem
  RESPIRATORY RHYTHM : Outport  InitialOutput=1.2221e-017
  Breathing_Enable : Outport  Port=2  InitialOutput=1.2221e-017
  tag scope: Breathing_Enable=global, Breathing_Frequency=global
  wires:
  D_Total/1 -> 60*TI/TT/1
  Variable Breathing Period Reset/1(Enable Breathing Signal) -> Enable Breathing Signal/1(Enable Breathing), Respiratory Rhythm_Generator/Enable
  Enable Breathing Signal/1(Enable_Breathing_Period) -> [Breathing_Enable], Breathing_Enable/1
  Variable Breathing Period Reset/2(Variable Breathing Period) -> Respiratory Rhythm_Generator/1(VBP Variable Breathing Period), Math Function/1
  Respiratory Rhythm_Generator/1(Respiratory Rhythm) -> RESPIRATORY RHYTHM/1  "Respiratory Rhythm (sec) INSPIRATION INTERVAL=EXPIRATION INTERVAL"
  Math Function/1 -> Gain/1
  Gain/1 -> [Breathing_Frequency]
  60*TI/TT/1 -> VBF_fcn/1
  VBF_fcn/1 -> Ventilator override/1(Central Respiration Rate)
  Ventilator override/1(Respiration Rate) -> Variable Breathing Period Reset/1(Breathing Freq (breaths/min))

== system PNEUMA/Central Neural Control/VENTILATORY DRIVE (chemical) ==
  SI : Inport
  PbCO2 : Inport  Port=2
  SAO2 : Inport  Port=3
  Sleep/Awake : Inport  Port=4
  AI : Inport  Port=5
  PaCO2 : Inport  Port=6
  " 1 for up 0 for ground" : Constant
  Dynamic Drive : Subsystem
  Fcn : Fcn  Expr=(u>0)*u
  Fcn1 : Fcn  Expr=(u>0)*u
  Fcn2 : Fcn  Expr=u(2)*(1-0.4*u(1))
  Gc : Gain  Gain=0.075  SaturateOnIntegerOverflow=on  OutDataTypeStr=Inherit: Same as input  ParamDataTypeStr=Inherit: Same as input
  Gc_blocker : Gain  SaturateOnIntegerOverflow=on  OutDataTypeStr=Inherit: Same as input  ParamDataTypeStr=Inherit: Same as input
  Gp : Gain  Gain=0.0063  SaturateOnIntegerOverflow=on  OutDataTypeStr=Inherit: Same as input  ParamDataTypeStr=Inherit: Same as input
  Gp_blocker : Gain  SaturateOnIntegerOverflow=on  OutDataTypeStr=Inherit: Same as input  ParamDataTypeStr=Inherit: Same as input
  Ic : Constant  Value=Ic
  IpCO2 : Constant  Value=IpCO2
  IpO2 : Constant  Value=IpO2
  Memory : Memory  InitialCondition=DtotalIC
  Mux3 : Mux
  Product : Product  InputSameDT=on  SaturateOnIntegerOverflow=on  OutDataTypeStr=Inherit: Same as first input
  S_wake : Gain  Gain=0.3  SaturateOnIntegerOverflow=on  OutDataTypeStr=Inherit: Same as input  ParamDataTypeStr=Inherit: Same as input
  Sum : Sum  InputSameDT=on  SaturateOnIntegerOverflow=on  OutDataTypeStr=Inherit: Same as first input
  Sum1 : Sum  Inputs=+-  InputSameDT=on  SaturateOnIntegerOverflow=on  OutDataTypeStr=Inherit: Same as first input
  Sum2 : Sum  Inputs=+-  InputSameDT=on  SaturateOnIntegerOverflow=on  OutDataTypeStr=Inherit: Same as first input
  Sum3 : Sum  Inputs=+-  InputSameDT=on  SaturateOnIntegerOverflow=on  OutDataTypeStr=Inherit: Same as first input
  Sum4 : Sum  Inputs=-+  InputSameDT=on  SaturateOnIntegerOverflow=on  OutDataTypeStr=Inherit: Same as first input
  Switch : Switch  Threshold=0.5  SaturateOnIntegerOverflow=off  InputSameDT=off
  D_Total : Outport
  tag scope: Dchemo=global
  wires:
  Gc_blocker/1 -> Fcn/1
  Product/1 -> Gp/1
  Fcn1/1 -> Sum/2
  Fcn/1 -> Sum/1
  SAO2/1 -> Sum2/2
  PaCO2/1 -> Sum3/1
  PbCO2/1 -> Sum1/1
  Ic/1 -> Sum1/2
  IpCO2/1 -> Sum3/2
  IpO2/1 -> Sum2/1
  Gc/1 -> Gc_blocker/1
  Sum1/1 -> Gc/1
  Gp_blocker/1 -> Fcn1/1
  Sum3/1 -> Product/1
  Sum2/1 -> Product/2
  Dynamic Drive/1(Out1) -> Switch/3
  Sum4/1 -> Mux3/2
  Fcn2/1 -> Memory/1
  Mux3/1 -> Fcn2/1
  Sum/1 -> [Dchemo], Sum4/2
  S_wake/1 -> Sum4/1
  Gp/1 -> Gp_blocker/1
  Memory/1 -> Switch/1, Dynamic Drive/1(In1)
  " 1 for up 0 for ground"/1 -> Switch/2
  Switch/1 -> D_Total/1
  Sleep/Awake/1 -> Mux3/3
  AI/1 -> Mux3/4
  SI/1 -> S_wake/1, Mux3/1

== system PNEUMA/Central Neural Control/Ventilator override ==
  Neural drive : Inport
  Divide : Product  Inputs=**
  "Modified drive " : Outport
  wires:
  [NeuroMuscleBlock] -> Divide/1
  Neural drive/1 -> Divide/2  "Neural drive"
  Divide/1 -> "Modified drive "/1

== system PNEUMA/Central Neural Control/chemoreflex ==
  PaO2 : Inport
  PaCO2 : Inport  Port=2
  1/tau_chemo : Gain  Gain=1/tau_chemo  SaturateOnIntegerOverflow=on  OutDataTypeStr=Inherit: Same as input  ParamDataTypeStr=Inherit: Same as input
  Fcn -23 blocks1 : Fcn  Expr=((u(1)<40) * ( K_H -1.6) + (u(1)>80) * K_H + ( K_H - (u(1) - 80) * (1.2/30)) * ( (u(1) >=40) && ( u(1)<=80) ) ) * (log(u(2) * 1/PaCO2_chemo_n) ) + f_chemo_co2_n
  Fcn -9 blocks : Fcn  Expr="(exp((u(2) - u(1) )* (1/kchemo))  *fchemo_min+ fchemo_max)/(exp((u(2) - u(1) )* (1/kchemo)) + 1)"
  Integrator : Integrator  InitialCondition=fchemoIC
  Mux : Mux  Inputs=2
  Mux1 : Mux  Inputs=2
  PaO2_chemo_n : Constant  Value=PaO2_chemo_n
  Product5 : Product  Inputs=**  InputSameDT=on  SaturateOnIntegerOverflow=on  OutDataTypeStr=Inherit: Same as first input
  Sum8 : Sum  Inputs=+-  InputSameDT=on  SaturateOnIntegerOverflow=on  OutDataTypeStr=Inherit: Same as first input
  f_chemo : Outport
  wires:
  PaO2_chemo_n/1 -> Mux/1
  PaO2/1 -> Mux/2, Mux1/1
  Fcn -9 blocks/1 -> Product5/1
  Fcn -23 blocks1/1 -> Product5/2
  Product5/1 -> Sum8/1
  Integrator/1 -> f_chemo/1, Sum8/2
  1/tau_chemo/1 -> Integrator/1
  Sum8/1 -> 1/tau_chemo/1
  Mux/1 -> Fcn -9 blocks/1
  Mux1/1 -> Fcn -23 blocks1/1
  PaCO2/1 -> Mux1/2

== system PNEUMA/Central Neural Control/lung feedback ==
  Vt : Inport
  1/tau_ls : Gain  Gain=1/tau_ls  SaturateOnIntegerOverflow=on  OutDataTypeStr=Inherit: Same as input  ParamDataTypeStr=Inherit: Same as input
  Abs1 : Abs  SaturateOnIntegerOverflow=off
  G_ls : Gain  Gain=Gls  SaturateOnIntegerOverflow=on  OutDataTypeStr=Inherit: Same as input  ParamDataTypeStr=Inherit: Same as input
  Integrator : Integrator  InitialCondition=flsIC
  Sum8 : Sum  Inputs=+-  InputSameDT=on  SaturateOnIntegerOverflow=on  OutDataTypeStr=Inherit: Same as first input
  lung firing saturation : Saturate  UpperLimit=100  LowerLimit=0
  f_ls : Outport
  wires:
  Vt/1 -> Abs1/1
  Sum8/1 -> 1/tau_ls/1
  1/tau_ls/1 -> Integrator/1
  Integrator/1 -> Sum8/2, lung firing saturation/1
  G_ls/1 -> Sum8/1
  Abs1/1 -> G_ls/1
  lung firing saturation/1 -> f_ls/1

== system PNEUMA/Display Panels/Saving CARDIORESPIRATORY ==
  In1 : Inport
  In2 : Inport  Port=2
  Clock : Clock
  Gain : Gain  Gain=1/(3600*24*DAY)
  If : If  IfExpression=(u1>777600)&(u1<=864000)  ShowElse=off
  If Action Subsystem : Subsystem  TreatAsAtomicUnit=on
  Rounding Function : Rounding
  Switch Case : SwitchCase  CaseConditions={0,1,2,3,4,5,6,7,8}  SampleTime=sampletime
  Switch Case Action Subsystem : Subsystem  TreatAsAtomicUnit=on
  Switch Case Action Subsystem1 : Subsystem  TreatAsAtomicUnit=on
  Switch Case Action Subsystem2 : Subsystem  TreatAsAtomicUnit=on
  Switch Case Action Subsystem3 : Subsystem  TreatAsAtomicUnit=on
  Switch Case Action Subsystem4 : Subsystem  TreatAsAtomicUnit=on
  Switch Case Action Subsystem5 : Subsystem  TreatAsAtomicUnit=on
  Switch Case Action Subsystem6 : Subsystem  TreatAsAtomicUnit=on
  Switch Case Action Subsystem7 : Subsystem  TreatAsAtomicUnit=on
  Switch Case Action Subsystem8 : Subsystem  TreatAsAtomicUnit=on
  Switch Case Action Subsystem9 : Subsystem  TreatAsAtomicUnit=on
  wires:
  Clock/1 -> Gain/1, If/1
  Switch Case/1 -> Switch Case Action Subsystem/Action
  Switch Case/2 -> Switch Case Action Subsystem1/Action
  Switch Case/3 -> Switch Case Action Subsystem2/Action
  Switch Case/10 -> Switch Case Action Subsystem3/Action
  Rounding Function/1 -> Switch Case/1
  In1/1 -> Switch Case Action Subsystem/1(In1), Switch Case Action Subsystem1/1(In1), Switch Case Action Subsystem2/1(In1), Switch Case Action Subsystem5/1(In1), Switch Case Action Subsystem3/1(In1), Switch Case Action Subsystem9/1(In1), Switch Case Action Subsystem8/1(In1), Switch Case Action Subsystem7/1(In1), Switch Case Action Subsystem6/1(In1), Switch Case Action Subsystem4/1(In1)
  Gain/1 -> Rounding Function/1
  Switch Case/4 -> Switch Case Action Subsystem4/Action
  Switch Case/5 -> Switch Case Action Subsystem5/Action
  Switch Case/6 -> Switch Case Action Subsystem6/Action
  Switch Case/7 -> Switch Case Action Subsystem7/Action
  Switch Case/8 -> Switch Case Action Subsystem8/Action
  Switch Case/9 -> Switch Case Action Subsystem9/Action
  If/1 -> If Action Subsystem/Action
  In2/1 -> If Action Subsystem/1(In1)

== system PNEUMA/Display Panels/Saving CARDIO ==
  In1 : Inport
  Clock : Clock
  Gain : Gain  Gain=1/(3600*24*DAY)
  Rounding Function : Rounding
  Switch Case : SwitchCase  CaseConditions={0,1,2,3,4,5,6,7,8}  SampleTime=sampletime
  Switch Case Action Subsystem : Subsystem  TreatAsAtomicUnit=on
  Switch Case Action Subsystem1 : Subsystem  TreatAsAtomicUnit=on
  Switch Case Action Subsystem2 : Subsystem  TreatAsAtomicUnit=on
  Switch Case Action Subsystem3 : Subsystem  TreatAsAtomicUnit=on
  Switch Case Action Subsystem4 : Subsystem  TreatAsAtomicUnit=on
  Switch Case Action Subsystem5 : Subsystem  TreatAsAtomicUnit=on
  Switch Case Action Subsystem6 : Subsystem  TreatAsAtomicUnit=on
  Switch Case Action Subsystem7 : Subsystem  TreatAsAtomicUnit=on
  Switch Case Action Subsystem8 : Subsystem  TreatAsAtomicUnit=on
  Switch Case Action Subsystem9 : Subsystem  TreatAsAtomicUnit=on
  wires:
  Clock/1 -> Gain/1
  Switch Case/1 -> Switch Case Action Subsystem/Action
  Switch Case/2 -> Switch Case Action Subsystem1/Action
  Switch Case/3 -> Switch Case Action Subsystem2/Action
  Switch Case/10 -> Switch Case Action Subsystem3/Action
  Rounding Function/1 -> Switch Case/1
  In1/1 -> Switch Case Action Subsystem/1(In1), Switch Case Action Subsystem1/1(In1), Switch Case Action Subsystem2/1(In1), Switch Case Action Subsystem5/1(In1), Switch Case Action Subsystem3/1(In1), Switch Case Action Subsystem9/1(In1), Switch Case Action Subsystem8/1(In1), Switch Case Action Subsystem7/1(In1), Switch Case Action Subsystem6/1(In1), Switch Case Action Subsystem4/1(In1)
  Gain/1 -> Rounding Function/1
  Switch Case/4 -> Switch Case Action Subsystem4/Action
  Switch Case/5 -> Switch Case Action Subsystem5/Action
  Switch Case/6 -> Switch Case Action Subsystem6/Action
  Switch Case/7 -> Switch Case Action Subsystem7/Action
  Switch Case/8 -> Switch Case Action Subsystem8/Action
  Switch Case/9 -> Switch Case Action Subsystem9/Action

== system PNEUMA/External Pressure/Annoxia or hypercapnia ==
  Divide : Product  Inputs=**
  Fcn1 : Fcn  Expr=1-1/(1+exp(-0.1*(u(1)-20)))^50
  Fcn2 : Fcn  Expr=(u(1)>PAO2IC)+(u(1)<=PAO2IC)*u(1)/PAO2IC
  Muscle_Contractility : Outport
  wires:
  Fcn2/1 -> Divide/1
  Fcn1/1 -> Divide/2
  [PaO2] -> Fcn2/1
  [PaCO2] -> Fcn1/1
  Divide/1 -> Muscle_Contractility/1

== system PNEUMA/External Pressure/CPAP Control ==
  Step : Step  Time=begin_time  Before=init_value  After=final_value  SampleTime=0
  Step1 : Step  Time=end_time  After=init_value-final_value  SampleTime=0
  Sum : Sum  Inputs=|++  InputSameDT=on  SaturateOnIntegerOverflow=on  OutDataTypeStr=Inherit: Same as first input
  Out1 : Outport
  wires:
  Sum/1 -> Out1/1
  Step1/1 -> Sum/2
  Step/1 -> Sum/1

== system PNEUMA/External Pressure/CPAP Pressure ==
  Step : Step  Time=begin_time  Before=init_value  After=final_value  SampleTime=0
  Step1 : Step  Time=end_time  After=init_value-final_value  SampleTime=0
  Sum : Sum  Inputs=|++  InputSameDT=on  SaturateOnIntegerOverflow=on  OutDataTypeStr=Inherit: Same as first input
  Out1 : Outport
  wires:
  Sum/1 -> Out1/1
  Step1/1 -> Sum/2
  Step/1 -> Sum/1
